simulink model "CM200A_DmaCfgAndUse"  (R2013b)
settings: Solver=ode1  StartTime=0.0  StopTime=Inf  FixedStep=0.001  RelTol=1e-3
values from neighbouring files (symbols this model uses):
  MOTAG0MEAS_MOTAG0READPTRRST_CNT_U32 = DataDict.Constant    [CM200A_DmaCfgAndUse_DataDict.m]
  MOTAG0MEAS_MOTAG0TRSMSTRTININ_CNT_U32 = DataDict.Constant    [CM200A_DmaCfgAndUse_DataDict.m]
  MOTAG1MEAS_MOTAG1READPTRRST_CNT_U32 = DataDict.Constant    [CM200A_DmaCfgAndUse_DataDict.m]
  MOTAG1MEAS_MOTAG1TRSMSTRTININ_CNT_U32 = DataDict.Constant    [CM200A_DmaCfgAndUse_DataDict.m]
libraries: simulink x1
settings Model: BufferReuse=off  Creator=Keyur Patel  LastModifiedBy=CZ68DS
settings OptimizationCC: BlockReduction=off  DefaultUnderspecifiedDataType=single  OptimizeBlockIOStorage=off  BufferReuse=off  ExpressionFolding=off  LocalBlockOutputs=off  OptimizeModelRefInitCode=on  LifeSpan=Inf
settings HardwareCC: ProdIntDivRoundTo=Zero  ProdEndianess=BigEndian  ProdHWDeviceType=Generic->Custom  TargetIntDivRoundTo=Zero  TargetEndianess=BigEndian  TargetHWDeviceType=Generic->Custom
settings RTWCC: SystemTargetFile=ert.tlc  TemplateMakefile=ert_default_tmf  Description=Embedded Coder  ProcessScript=ert_make_rtw_hook
settings CodeAppCC: IgnoreCustomStorageClasses=off
settings ERTTargetCC: CodeReplacementLibrary=ANSI_C  GenerateSampleERTMain=on  ERTCustomFileTemplate=example_file_process.tlc

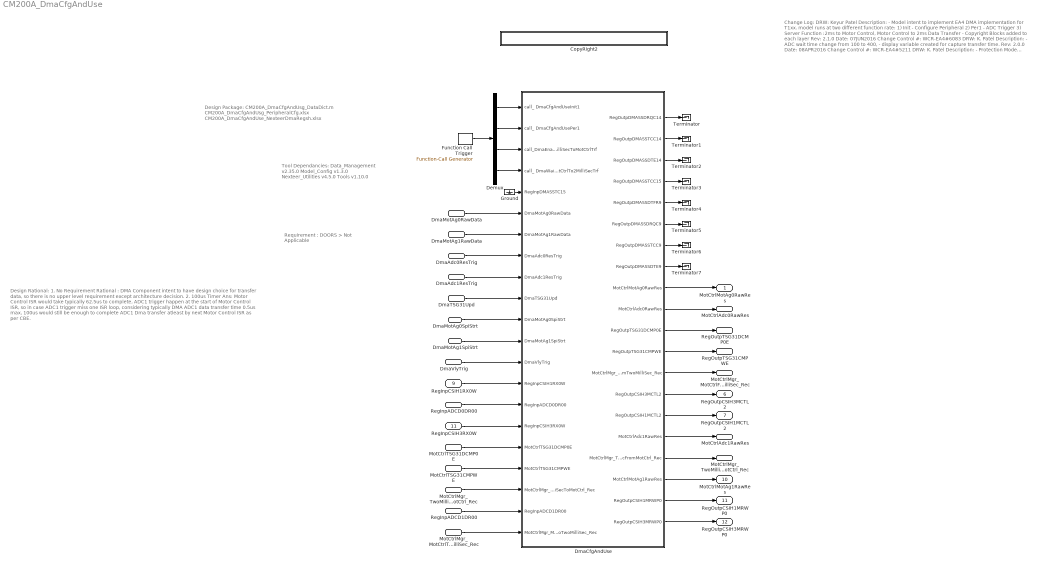
== system CM200A_DmaCfgAndUse ==
  note: Design Package:
      |
      | CM200A_DmaCfgAndUsg_DataDict.m
      | CM200A_DmaCfgAndUsg_PeripheralCfg.xlsx
      | CM200A_DmaCfgAndUse_NexteerDmaRegsh.xlsx
  note: Tool Dependancies:
      |
      | Data_Management v2.35.0
      | Model_Config v1.3.0
      | Nexteer_Utilities v4.5.0
      | Tools v1.10.0
  note: Requirement :
      |
      | DOORS > Not Applicable
  note: Change Log:
      |
      | DRW: Keyur Patel
      | Description:
      | - Model intent to implement EA4 DMA implementation for T1xx.
      |    model runs at two different function rate:
      |       1) Init - Configure Peripheral
      | 	 2) Per1 - ADC Trigger
      | 	 3) Server Function :2ms to Motor Control, Motor Control to 2ms Data Transfer
      | - Copyright Blocks added to each layer
      |
      | Rev: 2.1.0
      | Date: 07JUN2016
      | Change Control #: WCR-EA4#6083
      | DRW: K. Patel
      | Description:
      | - ADC wait time change from 100 to 400,
      | - display variable created for capture transfer time.
      |
      | Rev: 2.0.0
      | Date: 08APR2016
      | Change Control #: WCR-EA4#5211
      | DRW: K. Patel
      | Description:
      | - Protection Mode Change : change in "CM200A_DmaCfgAndUsg_PeripheralCfg.xlsx"
      |
      |
      | Rev: 1.5.0
      | Date: 21OCT2015
      | Change Control #: WCR-EA4#3226
      | DRW: Erlenbeck
      | Description:
      | -Added channels to reset the read pointers on the MotAg SPI peripherals
      |
      | Rev: 1.4.0
      | Date: 20OCT2015
      | Change Control #: WCR-EA4#1460
      | DRW: K. Patel
      | Description:
      | -DMA Channel Master Configuration change in "CM200A_DmaCfgAndUsg_PeripheralCfg.xlsx"
      |
      | Rev: 1.3.0
      | Date: 15JUL2015
      | Change Control #: WCR-EA4#1110
      | DRW: K. Patel
      | Description:
      | -Motor Angle 1 SPI Trigger from Valley Added
      |
      | Rev: 1.2.0
      | Date: 19JUN2015
      | Change Control #: WCR-EA4#861
      | DRW: K. Patel
      | Description:
      | -Rework (DMALOCALOFFSET constant)
      |
      |
      | Rev: 1.1.0
      | Date: 29APR2015
      | Change Control #: WCR-EA4#688
      | DRW: K. Patel
      | Description:
      | -Rework
      |
      | Rev: 1.0.0
      | Date: 29APR2015
      | Change Control #: WCR-EA4#407
      | DRW: K. Patel
      | Description:
      | - Initial Release
  note: Design Rational:
      | 1. No Requirement
      | Rational :  DMA Component intent to have design choice for transfer data, so there is no upper level
      | requirement except architecture decision.
      |
      | 2. 100us Timer
      | Ans: Motor Control ISR would take typically 62.5us to complete, ADC1 trigger happen at the start of Motor
      | Control ISR, so in case ADC1  trigger miss one ISR loop, considering typically DMA ADC1 data transfer time
      | 0.5us max, 100us would still be enough to complete ADC1 Dma transfer atleast by next Motor Control
      | ISR as per CBE.
  DmaMotAg0RawData : Inport
  DmaMotAg1RawData : Inport  Port=2
  DmaAdc0ResTrig : Inport  Port=3
  DmaAdc1ResTrig : Inport  Port=4
  DmaTSG31Upd : Inport  Port=5
  DmaMotAg0SpiStrt : Inport  Port=6
  DmaMotAg1SpiStrt : Inport  Port=7
  DmaVlyTrig : Inport  Port=8
  RegInpCSIH1RX0W : Inport  Description=DMA0-0 : Source Address  Port=9
  RegInpADCD0DR00 : Inport  Port=10
  RegInpCSIH3RX0W : Inport  Description=DMA0-0 : Source Address  Port=11
  MotCtrlTSG31DCMP0E : Inport  Description=DMA0-3 : Source Address  Port=12
  MotCtrlTSG31CMPWE : Inport  Description=DMA0-4 : Source Address  Port=13
  MotCtrlMgr_TwoMilliSecToMotCtrl_Rec : Inport  Description=DMA1-1 : Source Address  Port=14
  RegInpADCD1DR00 : Inport  Description=DMA1-6 : Source Address  Port=15
  MotCtrlMgr_MotCtrlToTwoMilliSec_Rec : Inport  Description=DMA1-7 : Source Address  Port=16
  CopyRight2 : Subsystem  Description=|  mask(Copyright Information){none=on}
      | Copyright info block.                                               
      |                                                                     
      | Place copyright information at the top of every subsystem in design.
      mask prompts: none "No parameters"
      mask help: Place copyright information at the top of every subsystem in design.
      mask Display:
      | NxtrConf = 'Nexteer Confidential';
      | 
      | sys = bdroot; %handle for the current model ("system")
      | first = get_param(sys,'Created');
      | first = first(end-3:end);  %year is last four digits
      | 
      | last = get_param(sys,'LastModifiedDate');
      | if isempty(last)
      |     last = datestr(now,'yyyy');
      | else
      |     last = last(end-3:end);
      | end
      | 
      | if strcmp(first,last)
      |     fprintf('%s -- Copyright %s Nexteer',NxtrConf,first)
      | else
      |     fprintf('%s -- %s%s- %s Nexteer',NxtrConf,char(169),first,last)
      | end
  Demux : Demux
  DmaCfgAndUse : Subsystem
  Function Call Trigger : simulink/Ports & Subsystems/Function-Call Generator  RequirementInfo="{'linktype_rmi_doors' '000089e3 (/E-STEER_New/System Specification Documents/Core Specs/Subsystem Specs/System Functions FDD/SF-46  Gross Cross Check)' '#211' 'true' 'REQ: SF046A_211' '' ; 'linktype_rmi_doors' '000089e3 (/E-STEER_New/System Specification Documents/Core Specs/Subsystem Specs/System Functions FDD/SF-46  Gross Cross Check)' '#182' 'true' 'REQ: SF046A_182' '' } %GIDa_688b36ec_1d40_4533_93c7_ec108d0c1aaf"  sample_time=0.002  numberOfIterations=1
  Ground : Ground
  Terminator{,1..7} (8 alike) : Terminator
  MotCtrlMotAg0RawRes : Outport  Description=DMA0-0: Destination Address
  MotCtrlAdc0RawRes : Outport  Description=DMA0-1: Destination Address  Port=2
  RegOutpTSG31DCMP0E : Outport  Description=DMA0-3: Destination Address  Port=3
  RegOutpTSG31CMPWE : Outport  Description=DMA0-4 : Destination Address  Port=4
  MotCtrlMgr_MotCtrlFromTwoMilliSec_Rec : Outport  Description=DMA1-1 : Destination Address  Port=5
  RegOutpCSIH3MCTL2 : Outport  Description=DMA1-4 : Destination Address  Port=6
  RegOutpCSIH1MCTL2 : Outport  Description=DMA1-4 : Destination Address  Port=7
  MotCtrlAdc1RawRes : Outport  Description=DMA1-6 : Destination Address  Port=8
  MotCtrlMgr_TwoMilliSecFromMotCtrl_Rec : Outport  Description=DMA1-7 : Destination Address  Port=9
  MotCtrlMotAg1RawRes : Outport  Description=DMA0-0: Destination Address  Port=10
  RegOutpCSIH1MRWP0 : Outport  Port=11
  RegOutpCSIH3MRWP0 : Outport  Port=12
      settings: AttributesFormatString=%<Description>
  wires:
  Function Call Trigger/1 -> Demux/1
  Demux/1 -> DmaCfgAndUse/1(call_ DmaCfgAndUseInit1)
  Demux/2 -> DmaCfgAndUse/2(call_ DmaCfgAndUsePer1)
  Demux/4 -> DmaCfgAndUse/4(call_ DmaWaitForMotCtrlTo2MilliSecTrf)
  Demux/3 -> DmaCfgAndUse/3(call_DmaEna2MilliSecToMotCtrlTrf)
  DmaCfgAndUse/1(RegOutpDMASSDRQC14) -> Terminator/1
  DmaCfgAndUse/2(RegOutpDMASSTCC14) -> Terminator1/1
  DmaCfgAndUse/3(RegOutpDMASSDTE14) -> Terminator2/1
  DmaCfgAndUse/7(RegOutpDMASSTCC9) -> Terminator6/1
  DmaCfgAndUse/6(RegOutpDMASSDRQC9) -> Terminator5/1
  DmaCfgAndUse/5(RegOutpDMASSDTFR9) -> Terminator4/1
  DmaCfgAndUse/8(RegOutpDMASSDTE9) -> Terminator7/1
  Ground/1 -> DmaCfgAndUse/5(RegInpDMASSTC15)
  DmaMotAg0RawData/1 -> DmaCfgAndUse/6(DmaMotAg0RawData)
  DmaAdc0ResTrig/1 -> DmaCfgAndUse/8(DmaAdc0ResTrig)
  DmaAdc1ResTrig/1 -> DmaCfgAndUse/9(DmaAdc1ResTrig)
  DmaTSG31Upd/1 -> DmaCfgAndUse/10(DmaTSG31Upd)
  DmaVlyTrig/1 -> DmaCfgAndUse/13(DmaVlyTrig)
  DmaMotAg0SpiStrt/1 -> DmaCfgAndUse/11(DmaMotAg0SpiStrt)
  DmaCfgAndUse/4(RegOutpDMASSTCC15) -> Terminator3/1
  RegInpADCD0DR00/1 -> DmaCfgAndUse/15(RegInpADCD0DR00)
  MotCtrlTSG31DCMP0E/1 -> DmaCfgAndUse/17(MotCtrlTSG31DCMP0E)
  MotCtrlTSG31CMPWE/1 -> DmaCfgAndUse/18(MotCtrlTSG31CMPWE)
  MotCtrlMgr_TwoMilliSecToMotCtrl_Rec/1 -> DmaCfgAndUse/19(MotCtrlMgr_TwoMilliSecToMotCtrl_Rec)
  RegInpADCD1DR00/1 -> DmaCfgAndUse/20(RegInpADCD1DR00)
  MotCtrlMgr_MotCtrlToTwoMilliSec_Rec/1 -> DmaCfgAndUse/21(MotCtrlMgr_MotCtrlToTwoMilliSec_Rec)
  DmaCfgAndUse/10(MotCtrlAdc0RawRes) -> MotCtrlAdc0RawRes/1
  DmaCfgAndUse/11(RegOutpTSG31DCMP0E) -> RegOutpTSG31DCMP0E/1
  DmaCfgAndUse/12(RegOutpTSG31CMPWE) -> RegOutpTSG31CMPWE/1
  DmaCfgAndUse/13(MotCtrlMgr_MotCtrlFromTwoMilliSec_Rec) -> MotCtrlMgr_MotCtrlFromTwoMilliSec_Rec/1
  DmaCfgAndUse/16(MotCtrlAdc1RawRes) -> MotCtrlAdc1RawRes/1
  DmaCfgAndUse/17(MotCtrlMgr_TwoMilliSecFromMotCtrl_Rec) -> MotCtrlMgr_TwoMilliSecFromMotCtrl_Rec/1
  RegInpCSIH1RX0W/1 -> DmaCfgAndUse/14(RegInpCSIH1RX0W)
  DmaCfgAndUse/15(RegOutpCSIH1MCTL2) -> RegOutpCSIH1MCTL2/1
  DmaCfgAndUse/9(MotCtrlMotAg0RawRes) -> MotCtrlMotAg0RawRes/1
  DmaMotAg1SpiStrt/1 -> DmaCfgAndUse/12(DmaMotAg1SpiStrt)
  DmaCfgAndUse/14(RegOutpCSIH3MCTL2) -> RegOutpCSIH3MCTL2/1
  RegInpCSIH3RX0W/1 -> DmaCfgAndUse/16(RegInpCSIH3RX0W)
  DmaCfgAndUse/18(MotCtrlMotAg1RawRes) -> MotCtrlMotAg1RawRes/1
  DmaMotAg1RawData/1 -> DmaCfgAndUse/7(DmaMotAg1RawData)
  DmaCfgAndUse/19(RegOutpCSIH1MRWP0) -> RegOutpCSIH1MRWP0/1
  DmaCfgAndUse/20(RegOutpCSIH3MRWP0) -> RegOutpCSIH3MRWP0/1

== system CM200A_DmaCfgAndUse/CopyRight2 ==

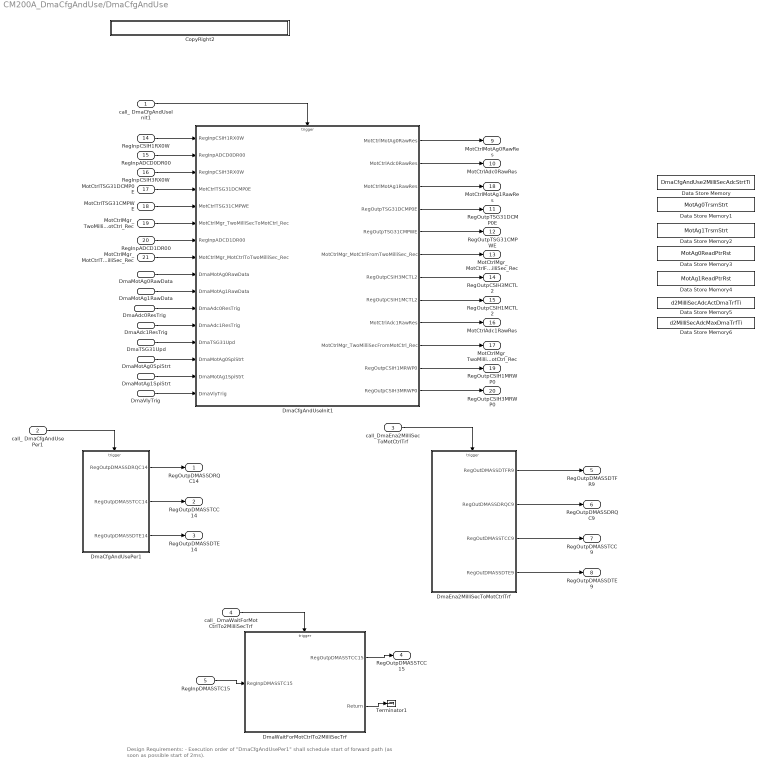
== system CM200A_DmaCfgAndUse/DmaCfgAndUse ==
  note: Design Requirements:
      |
      | - Execution order of "DmaCfgAndUsePer1" shall schedule start of forward path (as soon as possible start of 2ms).
  call_ DmaCfgAndUseInit1 : Inport
  call_ DmaCfgAndUsePer1 : Inport  Port=2
  call_DmaEna2MilliSecToMotCtrlTrf : Inport  Port=3
  call_ DmaWaitForMotCtrlTo2MilliSecTrf : Inport  Port=4
  RegInpDMASSTC15 : Inport  Port=5
  DmaMotAg0RawData : Inport  Description=Pysical Trigger: INTCSIH1IC1  Port=6
  DmaMotAg1RawData : Inport  Description=Pysical Trigger: INTCSIH1IC1  Port=7
  DmaAdc0ResTrig : Inport  Description=Physical Trigger : INTADCD0I3  Port=8
  DmaAdc1ResTrig : Inport  Description=Physical Trigger: INTADCD1I1  Port=9
  DmaTSG31Upd : Inport  Description=Physical Trigger: INTTSG31I11  Port=10
  DmaMotAg0SpiStrt : Inport  Description=Physical Trigger:INTTSG31I12  Port=11
  DmaMotAg1SpiStrt : Inport  Description=Physical Trigger:INTTSG31I12  Port=12
  DmaVlyTrig : Inport  Description=Physical Trigger: INTTSG31IVLY  Port=13
  RegInpCSIH1RX0W : Inport  Description=DMA0-0 : Source Address  Port=14
  RegInpADCD0DR00 : Inport  Port=15
  RegInpCSIH3RX0W : Inport  Description=DMA0-0 : Source Address  Port=16
  MotCtrlTSG31DCMP0E : Inport  Description=DMA0-3 : Source Address  Port=17
  MotCtrlTSG31CMPWE : Inport  Description=DMA0-4 : Source Address  Port=18
  MotCtrlMgr_TwoMilliSecToMotCtrl_Rec : Inport  Description=DMA1-1 : Source Address  Port=19
  RegInpADCD1DR00 : Inport  Description=DMA1-6 : Source Address  Port=20
  MotCtrlMgr_MotCtrlToTwoMilliSec_Rec : Inport  Description=DMA1-7 : Source Address  Port=21
  CopyRight2 : Subsystem  Description=|  mask(Copyright Information){none=on}
      | Copyright info block.                                               
      |                                                                     
      | Place copyright information at the top of every subsystem in design.
      mask prompts: none "No parameters"
      mask help: Place copyright information at the top of every subsystem in design.
      mask Display:
      | NxtrConf = 'Nexteer Confidential';
      | 
      | sys = bdroot; %handle for the current model ("system")
      | first = get_param(sys,'Created');
      | first = first(end-3:end);  %year is last four digits
      | 
      | last = get_param(sys,'LastModifiedDate');
      | if isempty(last)
      |     last = datestr(now,'yyyy');
      | else
      |     last = last(end-3:end);
      | end
      | 
      | if strcmp(first,last)
      |     fprintf('%s -- Copyright %s Nexteer',NxtrConf,first)
      | else
      |     fprintf('%s -- %s%s- %s Nexteer',NxtrConf,char(169),first,last)
      | end
  Data Store Memory : DataStoreMemory  DataStoreName=DmaCfgAndUse2MilliSecAdcStrtTi  ReadBeforeWriteMsg=warning  WriteAfterWriteMsg=warning  WriteAfterReadMsg=warning  StateMustResolveToSignalObject=on
  Data Store Memory1 : DataStoreMemory  DataStoreName=MotAg0TrsmStrt  ReadBeforeWriteMsg=warning  WriteAfterWriteMsg=warning  WriteAfterReadMsg=warning  StateMustResolveToSignalObject=on
  Data Store Memory2 : DataStoreMemory  DataStoreName=MotAg1TrsmStrt  ReadBeforeWriteMsg=warning  WriteAfterWriteMsg=warning  WriteAfterReadMsg=warning  StateMustResolveToSignalObject=on
  Data Store Memory3 : DataStoreMemory  DataStoreName=MotAg0ReadPtrRst  ReadBeforeWriteMsg=warning  WriteAfterWriteMsg=warning  WriteAfterReadMsg=warning  StateMustResolveToSignalObject=on
  Data Store Memory4 : DataStoreMemory  DataStoreName=MotAg1ReadPtrRst  ReadBeforeWriteMsg=warning  WriteAfterWriteMsg=warning  WriteAfterReadMsg=warning  StateMustResolveToSignalObject=on
  Data Store Memory5 : DataStoreMemory  DataStoreName=d2MilliSecAdcActDmaTrfTi  ReadBeforeWriteMsg=warning  WriteAfterWriteMsg=warning  WriteAfterReadMsg=warning  StateMustResolveToSignalObject=on
  Data Store Memory6 : DataStoreMemory  DataStoreName=d2MilliSecAdcMaxDmaTrfTi  ReadBeforeWriteMsg=warning  WriteAfterWriteMsg=warning  WriteAfterReadMsg=warning  StateMustResolveToSignalObject=on
  DmaCfgAndUseInit1 : Subsystem  TreatAsAtomicUnit=on
  DmaCfgAndUsePer1 : Subsystem  TreatAsAtomicUnit=on
  DmaEna2MilliSecToMotCtrlTrf : Subsystem  TreatAsAtomicUnit=on
  DmaWaitForMotCtrlTo2MilliSecTrf : Subsystem  TreatAsAtomicUnit=on
  Terminator1 : Terminator
  RegOutpDMASSDRQC14 : Outport
  RegOutpDMASSTCC14 : Outport  Port=2
  RegOutpDMASSDTE14 : Outport  Port=3
  RegOutpDMASSTCC15 : Outport  Port=4
  RegOutpDMASSDTFR9 : Outport  Port=5
  RegOutpDMASSDRQC9 : Outport  Port=6
  RegOutpDMASSTCC9 : Outport  Port=7
  RegOutpDMASSDTE9 : Outport  Port=8
  MotCtrlMotAg0RawRes : Outport  Description=DMA0-0: Destination Address  Port=9
  MotCtrlAdc0RawRes : Outport  Description=DMA0-1: Destination Address  Port=10
  RegOutpTSG31DCMP0E : Outport  Description=DMA0-3: Destination Address  Port=11
  RegOutpTSG31CMPWE : Outport  Description=DMA0-4 : Destination Address  Port=12
  MotCtrlMgr_MotCtrlFromTwoMilliSec_Rec : Outport  Description=DMA1-1 : Destination Address  Port=13
  RegOutpCSIH3MCTL2 : Outport  Description=DMA1-4 : Destination Address  Port=14
  RegOutpCSIH1MCTL2 : Outport  Description=DMA1-4 : Destination Address  Port=15
  MotCtrlAdc1RawRes : Outport  Description=DMA1-6 : Destination Address  Port=16
  MotCtrlMgr_TwoMilliSecFromMotCtrl_Rec : Outport  Description=DMA1-7 : Destination Address  Port=17
  MotCtrlMotAg1RawRes : Outport  Description=DMA0-0: Destination Address  Port=18
  RegOutpCSIH1MRWP0 : Outport  Port=19
  RegOutpCSIH3MRWP0 : Outport  Port=20
      settings: AttributesFormatString=%<Description>
  wires:
  call_ DmaCfgAndUseInit1/1 -> DmaCfgAndUseInit1/Trigger
  call_ DmaCfgAndUsePer1/1 -> DmaCfgAndUsePer1/Trigger
  call_ DmaWaitForMotCtrlTo2MilliSecTrf/1 -> DmaWaitForMotCtrlTo2MilliSecTrf/Trigger
  call_DmaEna2MilliSecToMotCtrlTrf/1 -> DmaEna2MilliSecToMotCtrlTrf/Trigger
  DmaCfgAndUsePer1/3(RegOutpDMASSDTE14) -> RegOutpDMASSDTE14/1
  DmaCfgAndUsePer1/2(RegOutpDMASSTCC14) -> RegOutpDMASSTCC14/1
  DmaCfgAndUsePer1/1(RegOutpDMASSDRQC14) -> RegOutpDMASSDRQC14/1
  DmaWaitForMotCtrlTo2MilliSecTrf/1(RegOutpDMASSTCC15) -> RegOutpDMASSTCC15/1
  DmaEna2MilliSecToMotCtrlTrf/2(RegOutDMASSDRQC9) -> RegOutpDMASSDRQC9/1
  DmaEna2MilliSecToMotCtrlTrf/4(RegOutDMASSDTE9) -> RegOutpDMASSDTE9/1
  DmaEna2MilliSecToMotCtrlTrf/3(RegOutDMASSTCC9) -> RegOutpDMASSTCC9/1
  DmaEna2MilliSecToMotCtrlTrf/1(RegOutDMASSDTFR9) -> RegOutpDMASSDTFR9/1
  RegInpDMASSTC15/1 -> DmaWaitForMotCtrlTo2MilliSecTrf/1(RegInpDMASSTC15)
  MotCtrlMgr_MotCtrlToTwoMilliSec_Rec/1 -> DmaCfgAndUseInit1/8(MotCtrlMgr_MotCtrlToTwoMilliSec_Rec)
  RegInpADCD0DR00/1 -> DmaCfgAndUseInit1/2(RegInpADCD0DR00)
  RegInpADCD1DR00/1 -> DmaCfgAndUseInit1/7(RegInpADCD1DR00)
  MotCtrlMgr_TwoMilliSecToMotCtrl_Rec/1 -> DmaCfgAndUseInit1/6(MotCtrlMgr_TwoMilliSecToMotCtrl_Rec)
  MotCtrlTSG31DCMP0E/1 -> DmaCfgAndUseInit1/4(MotCtrlTSG31DCMP0E)
  MotCtrlTSG31CMPWE/1 -> DmaCfgAndUseInit1/5(MotCtrlTSG31CMPWE)
  RegInpCSIH1RX0W/1 -> DmaCfgAndUseInit1/1(RegInpCSIH1RX0W)
  DmaMotAg0RawData/1 -> DmaCfgAndUseInit1/9(DmaMotAg0RawData)
  DmaAdc0ResTrig/1 -> DmaCfgAndUseInit1/11(DmaAdc0ResTrig)
  DmaAdc1ResTrig/1 -> DmaCfgAndUseInit1/12(DmaAdc1ResTrig)
  DmaTSG31Upd/1 -> DmaCfgAndUseInit1/13(DmaTSG31Upd)
  DmaMotAg0SpiStrt/1 -> DmaCfgAndUseInit1/14(DmaMotAg0SpiStrt)
  DmaVlyTrig/1 -> DmaCfgAndUseInit1/16(DmaVlyTrig)
  DmaWaitForMotCtrlTo2MilliSecTrf/2(Return) -> Terminator1/1
  DmaCfgAndUseInit1/2(MotCtrlAdc0RawRes) -> MotCtrlAdc0RawRes/1
  DmaCfgAndUseInit1/10(MotCtrlMgr_TwoMilliSecFromMotCtrl_Rec) -> MotCtrlMgr_TwoMilliSecFromMotCtrl_Rec/1
  DmaCfgAndUseInit1/1(MotCtrlMotAg0RawRes) -> MotCtrlMotAg0RawRes/1
  DmaCfgAndUseInit1/4(RegOutpTSG31DCMP0E) -> RegOutpTSG31DCMP0E/1
  DmaCfgAndUseInit1/5(RegOutpTSG31CMPWE) -> RegOutpTSG31CMPWE/1
  DmaCfgAndUseInit1/9(MotCtrlAdc1RawRes) -> MotCtrlAdc1RawRes/1
  DmaCfgAndUseInit1/6(MotCtrlMgr_MotCtrlFromTwoMilliSec_Rec) -> MotCtrlMgr_MotCtrlFromTwoMilliSec_Rec/1
  DmaCfgAndUseInit1/8(RegOutpCSIH1MCTL2) -> RegOutpCSIH1MCTL2/1
  DmaMotAg1SpiStrt/1 -> DmaCfgAndUseInit1/15(DmaMotAg1SpiStrt)
  DmaCfgAndUseInit1/7(RegOutpCSIH3MCTL2) -> RegOutpCSIH3MCTL2/1
  RegInpCSIH3RX0W/1 -> DmaCfgAndUseInit1/3(RegInpCSIH3RX0W)
  DmaCfgAndUseInit1/3(MotCtrlMotAg1RawRes) -> MotCtrlMotAg1RawRes/1
  DmaMotAg1RawData/1 -> DmaCfgAndUseInit1/10(DmaMotAg1RawData)
  DmaCfgAndUseInit1/11(RegOutpCSIH1MRWP0) -> RegOutpCSIH1MRWP0/1
  DmaCfgAndUseInit1/12(RegOutpCSIH3MRWP0) -> RegOutpCSIH3MRWP0/1

== system CM200A_DmaCfgAndUse/DmaCfgAndUse/CopyRight2 ==

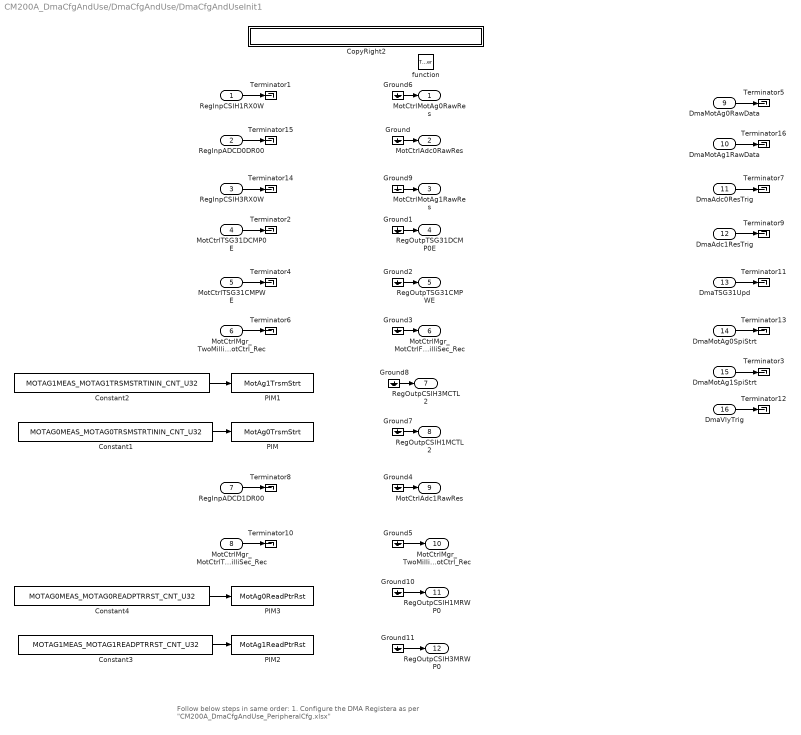
== system CM200A_DmaCfgAndUse/DmaCfgAndUse/DmaCfgAndUseInit1 ==
  note: Follow below steps in same order:
      |
      | 1. Configure the DMA Registera as per  "CM200A_DmaCfgAndUse_PeripheralCfg.xlsx"
  RegInpCSIH1RX0W : Inport  Description=DMA0-0 : Source Address
      settings: AttributesFormatString=%<Description>
  RegInpADCD0DR00 : Inport  Port=2
      settings: AttributesFormatString=DMA0-1 : Source Address
  RegInpCSIH3RX0W : Inport  Description=DMA0-2 : Source Address  Port=3
      settings: AttributesFormatString=%<Description>
  MotCtrlTSG31DCMP0E : Inport  Port=4
      settings: AttributesFormatString=DMA0-3 : Source Address
  MotCtrlTSG31CMPWE : Inport  Port=5
      settings: AttributesFormatString=DMA0-4 : Source Address
  MotCtrlMgr_TwoMilliSecToMotCtrl_Rec : Inport  Port=6
      settings: AttributesFormatString=DMA1-1 : Source Address
  RegInpADCD1DR00 : Inport  Port=7
      settings: AttributesFormatString=DMA1-6 : Source Address
  MotCtrlMgr_MotCtrlToTwoMilliSec_Rec : Inport  Port=8
      settings: AttributesFormatString=DMA1-7 : Source Address
  DmaMotAg0RawData : Inport  Description=Pysical Trigger: INTCSIH1IC1  Port=9
      settings: AttributesFormatString=%<Description>
  DmaMotAg1RawData : Inport  Description=Pysical Trigger: INTCSIH3IC0  Port=10
      settings: AttributesFormatString=%<Description>
  DmaAdc0ResTrig : Inport  Description=Physical Trigger : INTADCD0I3  Port=11
      settings: AttributesFormatString=%<Description>
  DmaAdc1ResTrig : Inport  Description=Physical Trigger: INTADCD1I1  Port=12
      settings: AttributesFormatString=%<Description>
  DmaTSG31Upd : Inport  Description=Physical Trigger: INTTSG31I11  Port=13
      settings: AttributesFormatString=%<Description>
  DmaMotAg0SpiStrt : Inport  Description=Physical Trigger:INTTSG31I12  Port=14
      settings: AttributesFormatString=%<Description>
  DmaMotAg1SpiStrt : Inport  Description=Physical Trigger:INTTSG31VI  Port=15
      settings: AttributesFormatString=%<Description>
  DmaVlyTrig : Inport  Description=Physical Trigger: INTTSG31VI  Port=16
      settings: AttributesFormatString=%<Description>
  function : TriggerPort  TriggerType=function-call
  Constant1 : Constant  Value=MOTAG0MEAS_MOTAG0TRSMSTRTININ_CNT_U32
  Constant2 : Constant  Value=MOTAG1MEAS_MOTAG1TRSMSTRTININ_CNT_U32
  Constant3 : Constant  Value=MOTAG1MEAS_MOTAG1READPTRRST_CNT_U32
  Constant4 : Constant  Value=MOTAG0MEAS_MOTAG0READPTRRST_CNT_U32
  CopyRight2 : Subsystem  Description=|  mask(Copyright Information){none=on}
      | Copyright info block.                                               
      |                                                                     
      | Place copyright information at the top of every subsystem in design.
      mask prompts: none "No parameters"
      mask help: Place copyright information at the top of every subsystem in design.
      mask Display:
      | NxtrConf = 'Nexteer Confidential';
      | 
      | sys = bdroot; %handle for the current model ("system")
      | first = get_param(sys,'Created');
      | first = first(end-3:end);  %year is last four digits
      | 
      | last = get_param(sys,'LastModifiedDate');
      | if isempty(last)
      |     last = datestr(now,'yyyy');
      | else
      |     last = last(end-3:end);
      | end
      | 
      | if strcmp(first,last)
      |     fprintf('%s -- Copyright %s Nexteer',NxtrConf,first)
      | else
      |     fprintf('%s -- %s%s- %s Nexteer',NxtrConf,char(169),first,last)
      | end
  Ground{,1..11} (12 alike) : Ground
  PIM : DataStoreWrite  Description=DMA1-4 : Source Address  DataStoreName=MotAg0TrsmStrt
      settings: AttributesFormatString=%<Description>
  PIM1 : DataStoreWrite  Description=DMA1-2 : Source Address  DataStoreName=MotAg1TrsmStrt
      settings: AttributesFormatString=%<Description>
  PIM2 : DataStoreWrite  Description=DMA1-3 : Source Address  DataStoreName=MotAg1ReadPtrRst
      settings: AttributesFormatString=%<Description>
  PIM3 : DataStoreWrite  Description=DMA1-5 : Source Address  DataStoreName=MotAg0ReadPtrRst
      settings: AttributesFormatString=%<Description>
  Terminator{1..16} (16 alike) : Terminator
  MotCtrlMotAg0RawRes : Outport  Description=DMA0-0: Destination Address
      settings: AttributesFormatString=%<Description>
  MotCtrlAdc0RawRes : Outport  Description=DMA0-1: Destination Address  Port=2
      settings: AttributesFormatString=%<Description>
  MotCtrlMotAg1RawRes : Outport  Description=DMA0-2: Destination Address  Port=3
      settings: AttributesFormatString=%<Description>
  RegOutpTSG31DCMP0E : Outport  Description=DMA0-3: Destination Address  Port=4
      settings: AttributesFormatString=%<Description>
  RegOutpTSG31CMPWE : Outport  Description=DMA0-4 : Destination Address  Port=5
      settings: AttributesFormatString=%<Description>
  MotCtrlMgr_MotCtrlFromTwoMilliSec_Rec : Outport  Description=DMA1-1 : Destination Address  Port=6
      settings: AttributesFormatString=%<Description>
  RegOutpCSIH3MCTL2 : Outport  Description=DMA1-2 : Destination Address  Port=7
      settings: AttributesFormatString=%<Description>
  RegOutpCSIH1MCTL2 : Outport  Description=DMA1-4 : Destination Address  Port=8
      settings: AttributesFormatString=%<Description>
  MotCtrlAdc1RawRes : Outport  Description=DMA1-6 : Destination Address  Port=9
      settings: AttributesFormatString=%<Description>
  MotCtrlMgr_TwoMilliSecFromMotCtrl_Rec : Outport  Description=DMA1-7 : Destination Address  Port=10
      settings: AttributesFormatString=%<Description>
  RegOutpCSIH1MRWP0 : Outport  Description=DMA1-5 : Destination Address  Port=11
      settings: AttributesFormatString=%<Description>
  RegOutpCSIH3MRWP0 : Outport  Description=DMA1-3 : Destination Address  Port=12
      settings: AttributesFormatString=%<Description>
  wires:
  RegInpADCD0DR00/1 -> Terminator15/1
  MotCtrlTSG31DCMP0E/1 -> Terminator2/1
  MotCtrlTSG31CMPWE/1 -> Terminator4/1
  MotCtrlMgr_TwoMilliSecToMotCtrl_Rec/1 -> Terminator6/1
  RegInpADCD1DR00/1 -> Terminator8/1
  MotCtrlMgr_MotCtrlToTwoMilliSec_Rec/1 -> Terminator10/1
  Ground/1 -> MotCtrlAdc0RawRes/1
  Ground1/1 -> RegOutpTSG31DCMP0E/1
  Ground2/1 -> RegOutpTSG31CMPWE/1
  Ground3/1 -> MotCtrlMgr_MotCtrlFromTwoMilliSec_Rec/1
  Ground4/1 -> MotCtrlAdc1RawRes/1
  Ground5/1 -> MotCtrlMgr_TwoMilliSecFromMotCtrl_Rec/1
  RegInpCSIH1RX0W/1 -> Terminator1/1
  Ground6/1 -> MotCtrlMotAg0RawRes/1
  Ground7/1 -> RegOutpCSIH1MCTL2/1
  DmaMotAg0RawData/1 -> Terminator5/1
  DmaAdc0ResTrig/1 -> Terminator7/1
  DmaAdc1ResTrig/1 -> Terminator9/1
  DmaTSG31Upd/1 -> Terminator11/1
  DmaVlyTrig/1 -> Terminator12/1
  DmaMotAg0SpiStrt/1 -> Terminator13/1
  Constant1/1 -> PIM/1
  Ground8/1 -> RegOutpCSIH3MCTL2/1
  Constant2/1 -> PIM1/1
  DmaMotAg1SpiStrt/1 -> Terminator3/1
  RegInpCSIH3RX0W/1 -> Terminator14/1
  Ground9/1 -> MotCtrlMotAg1RawRes/1
  DmaMotAg1RawData/1 -> Terminator16/1
  Ground10/1 -> RegOutpCSIH1MRWP0/1
  Ground11/1 -> RegOutpCSIH3MRWP0/1
  Constant3/1 -> PIM2/1
  Constant4/1 -> PIM3/1

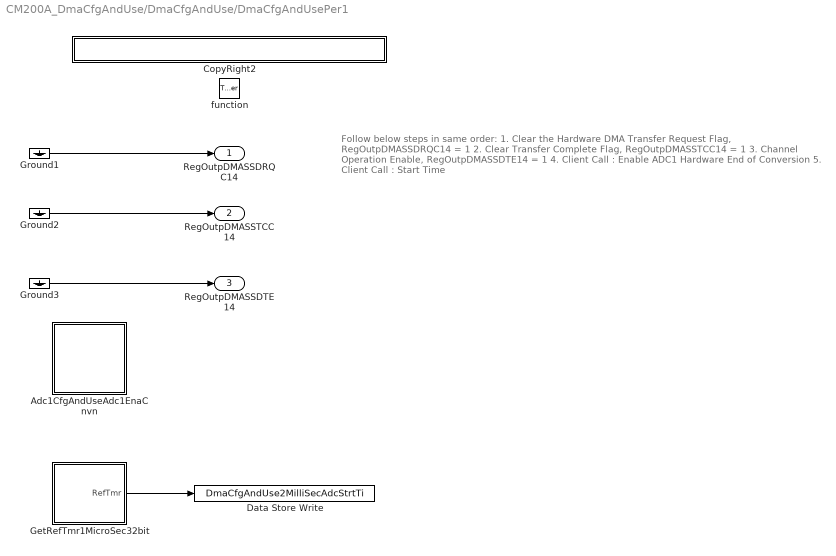
== system CM200A_DmaCfgAndUse/DmaCfgAndUse/DmaCfgAndUsePer1 ==
  note: Follow below steps in same order:
      |
      | 1. Clear the Hardware DMA Transfer Request Flag, RegOutpDMASSDRQC14 = 1
      | 2. Clear Transfer Complete Flag, RegOutpDMASSTCC14 = 1
      | 3. Channel Operation Enable, RegOutpDMASSDTE14 = 1
      | 4. Client Call : Enable ADC1 Hardware End of Conversion
      | 5. Client Call : Start Time
  function : TriggerPort  TriggerType=function-call
  Adc1CfgAndUseAdc1EnaCnvn : Subsystem
      settings: AttributesFormatString=Client Call : Enable ADC1 Hardware End of Conversion
  CopyRight2 : Subsystem  Description=|  mask(Copyright Information){none=on}
      | Copyright info block.                                               
      |                                                                     
      | Place copyright information at the top of every subsystem in design.
      mask prompts: none "No parameters"
      mask help: Place copyright information at the top of every subsystem in design.
      mask Display:
      | NxtrConf = 'Nexteer Confidential';
      | 
      | sys = bdroot; %handle for the current model ("system")
      | first = get_param(sys,'Created');
      | first = first(end-3:end);  %year is last four digits
      | 
      | last = get_param(sys,'LastModifiedDate');
      | if isempty(last)
      |     last = datestr(now,'yyyy');
      | else
      |     last = last(end-3:end);
      | end
      | 
      | if strcmp(first,last)
      |     fprintf('%s -- Copyright %s Nexteer',NxtrConf,first)
      | else
      |     fprintf('%s -- %s%s- %s Nexteer',NxtrConf,char(169),first,last)
      | end
  Data Store Write : DataStoreWrite  DataStoreName=DmaCfgAndUse2MilliSecAdcStrtTi
  GetRefTmr1MicroSec32bit : Subsystem
      settings: AttributesFormatString=Client Call : Start Time
  Ground1 : Ground
  Ground2 : Ground
  Ground3 : Ground
  RegOutpDMASSDRQC14 : Outport
  RegOutpDMASSTCC14 : Outport  Port=2
  RegOutpDMASSDTE14 : Outport  Port=3
  wires:
  Ground1/1 -> RegOutpDMASSDRQC14/1
  Ground2/1 -> RegOutpDMASSTCC14/1
  Ground3/1 -> RegOutpDMASSDTE14/1
  GetRefTmr1MicroSec32bit/1(RefTmr) -> Data Store Write/1

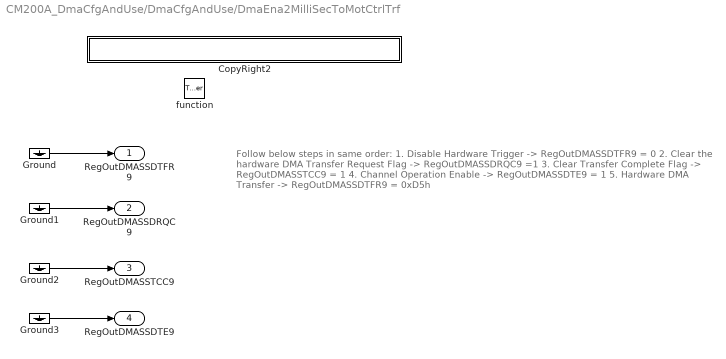
== system CM200A_DmaCfgAndUse/DmaCfgAndUse/DmaEna2MilliSecToMotCtrlTrf ==
  note: Follow below steps in same order:
      |
      | 1. Disable Hardware Trigger -> RegOutDMASSDTFR9 = 0
      | 2. Clear the hardware DMA Transfer Request Flag -> RegOutDMASSDRQC9 =1
      | 3. Clear Transfer Complete Flag -> RegOutDMASSTCC9 = 1
      | 4. Channel Operation Enable -> RegOutDMASSDTE9 = 1
      | 5. Hardware DMA Transfer -> RegOutDMASSDTFR9 = 0xD5h
  function : TriggerPort  TriggerType=function-call
  CopyRight2 : Subsystem  Description=|  mask(Copyright Information){none=on}
      | Copyright info block.                                               
      |                                                                     
      | Place copyright information at the top of every subsystem in design.
      mask prompts: none "No parameters"
      mask help: Place copyright information at the top of every subsystem in design.
      mask Display:
      | NxtrConf = 'Nexteer Confidential';
      | 
      | sys = bdroot; %handle for the current model ("system")
      | first = get_param(sys,'Created');
      | first = first(end-3:end);  %year is last four digits
      | 
      | last = get_param(sys,'LastModifiedDate');
      | if isempty(last)
      |     last = datestr(now,'yyyy');
      | else
      |     last = last(end-3:end);
      | end
      | 
      | if strcmp(first,last)
      |     fprintf('%s -- Copyright %s Nexteer',NxtrConf,first)
      | else
      |     fprintf('%s -- %s%s- %s Nexteer',NxtrConf,char(169),first,last)
      | end
  Ground{,1..3} (4 alike) : Ground
  RegOutDMASSDTFR9 : Outport
  RegOutDMASSDRQC9 : Outport  Port=2
  RegOutDMASSTCC9 : Outport  Port=3
  RegOutDMASSDTE9 : Outport  Port=4
  wires:
  Ground/1 -> RegOutDMASSDTFR9/1
  Ground1/1 -> RegOutDMASSDRQC9/1
  Ground2/1 -> RegOutDMASSTCC9/1
  Ground3/1 -> RegOutDMASSDTE9/1

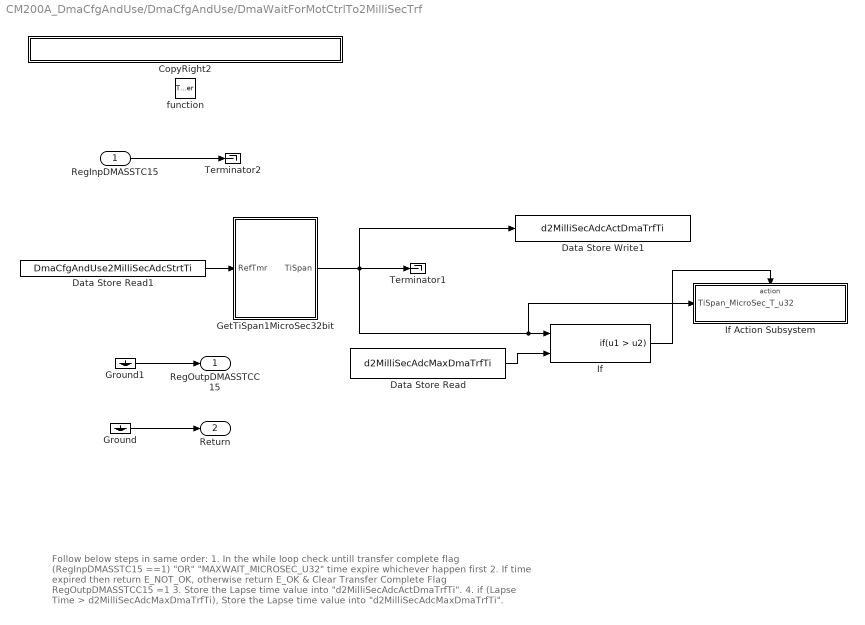
== system CM200A_DmaCfgAndUse/DmaCfgAndUse/DmaWaitForMotCtrlTo2MilliSecTrf ==
  note: Follow below steps in same order:
      |
      | 1. In the while loop check untill transfer complete flag (RegInpDMASSTC15 ==1) "OR" "MAXWAIT_MICROSEC_U32" time expire whichever happen first
      | 2. If time expired then return E_NOT_OK,
      |     otherwise return E_OK & Clear Transfer Complete Flag RegOutpDMASSTCC15 =1
      | 3. Store the Lapse time value into "d2MilliSecAdcActDmaTrfTi".
      | 4. if (Lapse Time > d2MilliSecAdcMaxDmaTrfTi), Store the Lapse time value into "d2MilliSecAdcMaxDmaTrfTi".
  RegInpDMASSTC15 : Inport
      settings: AttributesFormatString=Transfer Complete Flag Status Check
  function : TriggerPort  TriggerType=function-call
  CopyRight2 : Subsystem  Description=|  mask(Copyright Information){none=on}
      | Copyright info block.                                               
      |                                                                     
      | Place copyright information at the top of every subsystem in design.
      mask prompts: none "No parameters"
      mask help: Place copyright information at the top of every subsystem in design.
      mask Display:
      | NxtrConf = 'Nexteer Confidential';
      | 
      | sys = bdroot; %handle for the current model ("system")
      | first = get_param(sys,'Created');
      | first = first(end-3:end);  %year is last four digits
      | 
      | last = get_param(sys,'LastModifiedDate');
      | if isempty(last)
      |     last = datestr(now,'yyyy');
      | else
      |     last = last(end-3:end);
      | end
      | 
      | if strcmp(first,last)
      |     fprintf('%s -- Copyright %s Nexteer',NxtrConf,first)
      | else
      |     fprintf('%s -- %s%s- %s Nexteer',NxtrConf,char(169),first,last)
      | end
  Data Store Read : DataStoreRead  DataStoreName=d2MilliSecAdcMaxDmaTrfTi
  Data Store Read1 : DataStoreRead  DataStoreName=DmaCfgAndUse2MilliSecAdcStrtTi
  Data Store Write1 : DataStoreWrite  DataStoreName=d2MilliSecAdcActDmaTrfTi
  GetTiSpan1MicroSec32bit : Subsystem
  Ground : Ground
  Ground1 : Ground
  If : If  NumInputs=2  IfExpression=u1 > u2  ShowElse=off
  If Action Subsystem : Subsystem  TreatAsAtomicUnit=on
  Terminator1 : Terminator
      settings: Description=TiSpan_MicroSec_T_u32  AttributesFormatString=%<Description>
  Terminator2 : Terminator
  RegOutpDMASSTCC15 : Outport
  Return : Outport  Port=2
  wires:
  Ground1/1 -> RegOutpDMASSTCC15/1
  RegInpDMASSTC15/1 -> Terminator2/1
  Ground/1 -> Return/1
  Data Store Read1/1 -> GetTiSpan1MicroSec32bit/1(RefTmr)
  GetTiSpan1MicroSec32bit/1(TiSpan) -> Data Store Write1/1, If Action Subsystem/1(TiSpan_MicroSec_T_u32), If/1, Terminator1/1
  If/1 -> If Action Subsystem/Action
  Data Store Read/1 -> If/2

== system CM200A_DmaCfgAndUse/DmaCfgAndUse/DmaCfgAndUseInit1/CopyRight2 ==

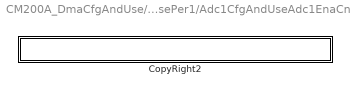
== system CM200A_DmaCfgAndUse/DmaCfgAndUse/DmaCfgAndUsePer1/Adc1CfgAndUseAdc1EnaCnvn ==
  CopyRight2 : Subsystem  Description=|  mask(Copyright Information){none=on}
      | Copyright info block.                                               
      |                                                                     
      | Place copyright information at the top of every subsystem in design.
      mask prompts: none "No parameters"
      mask help: Place copyright information at the top of every subsystem in design.
      mask Display:
      | NxtrConf = 'Nexteer Confidential';
      | 
      | sys = bdroot; %handle for the current model ("system")
      | first = get_param(sys,'Created');
      | first = first(end-3:end);  %year is last four digits
      | 
      | last = get_param(sys,'LastModifiedDate');
      | if isempty(last)
      |     last = datestr(now,'yyyy');
      | else
      |     last = last(end-3:end);
      | end
      | 
      | if strcmp(first,last)
      |     fprintf('%s -- Copyright %s Nexteer',NxtrConf,first)
      | else
      |     fprintf('%s -- %s%s- %s Nexteer',NxtrConf,char(169),first,last)
      | end

== system CM200A_DmaCfgAndUse/DmaCfgAndUse/DmaCfgAndUsePer1/CopyRight2 ==

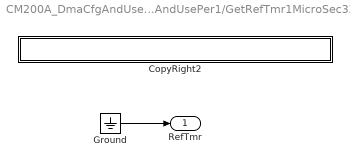
== system CM200A_DmaCfgAndUse/DmaCfgAndUse/DmaCfgAndUsePer1/GetRefTmr1MicroSec32bit ==
  CopyRight2 : Subsystem  Description=|  mask(Copyright Information){none=on}
      | Copyright info block.                                               
      |                                                                     
      | Place copyright information at the top of every subsystem in design.
      mask prompts: none "No parameters"
      mask help: Place copyright information at the top of every subsystem in design.
      mask Display:
      | NxtrConf = 'Nexteer Confidential';
      | 
      | sys = bdroot; %handle for the current model ("system")
      | first = get_param(sys,'Created');
      | first = first(end-3:end);  %year is last four digits
      | 
      | last = get_param(sys,'LastModifiedDate');
      | if isempty(last)
      |     last = datestr(now,'yyyy');
      | else
      |     last = last(end-3:end);
      | end
      | 
      | if strcmp(first,last)
      |     fprintf('%s -- Copyright %s Nexteer',NxtrConf,first)
      | else
      |     fprintf('%s -- %s%s- %s Nexteer',NxtrConf,char(169),first,last)
      | end
  Ground : Ground
  RefTmr : Outport
  wires:
  Ground/1 -> RefTmr/1

== system CM200A_DmaCfgAndUse/DmaCfgAndUse/DmaEna2MilliSecToMotCtrlTrf/CopyRight2 ==

== system CM200A_DmaCfgAndUse/DmaCfgAndUse/DmaWaitForMotCtrlTo2MilliSecTrf/CopyRight2 ==

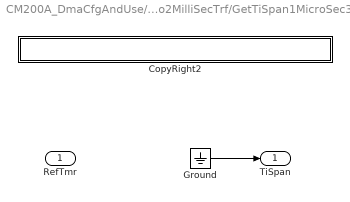
== system CM200A_DmaCfgAndUse/DmaCfgAndUse/DmaWaitForMotCtrlTo2MilliSecTrf/GetTiSpan1MicroSec32bit ==
  RefTmr : Inport
  CopyRight2 : Subsystem  Description=|  mask(Copyright Information){none=on}
      | Copyright info block.                                               
      |                                                                     
      | Place copyright information at the top of every subsystem in design.
      mask prompts: none "No parameters"
      mask help: Place copyright information at the top of every subsystem in design.
      mask Display:
      | NxtrConf = 'Nexteer Confidential';
      | 
      | sys = bdroot; %handle for the current model ("system")
      | first = get_param(sys,'Created');
      | first = first(end-3:end);  %year is last four digits
      | 
      | last = get_param(sys,'LastModifiedDate');
      | if isempty(last)
      |     last = datestr(now,'yyyy');
      | else
      |     last = last(end-3:end);
      | end
      | 
      | if strcmp(first,last)
      |     fprintf('%s -- Copyright %s Nexteer',NxtrConf,first)
      | else
      |     fprintf('%s -- %s%s- %s Nexteer',NxtrConf,char(169),first,last)
      | end
  Ground : Ground
  TiSpan : Outport
  wires:
  Ground/1 -> TiSpan/1

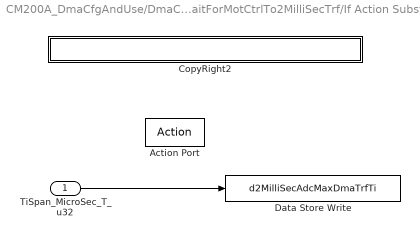
== system CM200A_DmaCfgAndUse/DmaCfgAndUse/DmaWaitForMotCtrlTo2MilliSecTrf/If Action Subsystem ==
  TiSpan_MicroSec_T_u32 : Inport
  Action Port : ActionPort  ActionType=then
  CopyRight2 : Subsystem  Description=|  mask(Copyright Information){none=on}
      | Copyright info block.                                               
      |                                                                     
      | Place copyright information at the top of every subsystem in design.
      mask prompts: none "No parameters"
      mask help: Place copyright information at the top of every subsystem in design.
      mask Display:
      | NxtrConf = 'Nexteer Confidential';
      | 
      | sys = bdroot; %handle for the current model ("system")
      | first = get_param(sys,'Created');
      | first = first(end-3:end);  %year is last four digits
      | 
      | last = get_param(sys,'LastModifiedDate');
      | if isempty(last)
      |     last = datestr(now,'yyyy');
      | else
      |     last = last(end-3:end);
      | end
      | 
      | if strcmp(first,last)
      |     fprintf('%s -- Copyright %s Nexteer',NxtrConf,first)
      | else
      |     fprintf('%s -- %s%s- %s Nexteer',NxtrConf,char(169),first,last)
      | end
  Data Store Write : DataStoreWrite  DataStoreName=d2MilliSecAdcMaxDmaTrfTi
  wires:
  TiSpan_MicroSec_T_u32/1 -> Data Store Write/1

== system CM200A_DmaCfgAndUse/DmaCfgAndUse/DmaCfgAndUsePer1/Adc1CfgAndUseAdc1EnaCnvn/CopyRight2 ==

== system CM200A_DmaCfgAndUse/DmaCfgAndUse/DmaCfgAndUsePer1/GetRefTmr1MicroSec32bit/CopyRight2 ==

== system CM200A_DmaCfgAndUse/DmaCfgAndUse/DmaWaitForMotCtrlTo2MilliSecTrf/GetTiSpan1MicroSec32bit/CopyRight2 ==

== system CM200A_DmaCfgAndUse/DmaCfgAndUse/DmaWaitForMotCtrlTo2MilliSecTrf/If Action Subsystem/CopyRight2 ==
